simulink model "PID_Simulation_System"  (R2018b)
settings: Solver=VariableStepAuto  StartTime=0.0  StopTime=30  RelTol=1e-3
values from neighbouring files (symbols this model uses):
  h = 5e-3    (= 0.005)    [main.m]
  k_noise = 1    [main.m]
  k_pertub = 1    [main.m]
  kd = 40    [main.m]
  ki = 180    [main.m]
  kp = 497    [main.m]
  p1 = -0.1    [Calc_Aux.m]    (also in main.m = poles(1))
  p2 = poles(2)    [main.m]
  Pertub = 1    [main.m]
  t_pertub = 5    [main.m]
undefined symbols (not defined in the file or in its folder): k
settings Model: Creator=fred  LastModifiedBy=root
settings HardwareCC: ProdBitPerLong=64  ProdHWDeviceType=Intel->x86-64 (Linux 64)

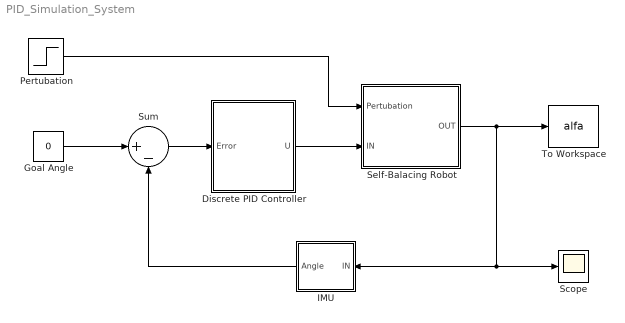
== system PID_Simulation_System ==
  Discrete PID Controller : Subsystem
  Goal Angle : Constant  Value=0
  IMU : Subsystem
  Pertubation : Step  Time=t_pertub  After=Pertub  SampleTime=h
  Scope : Scope
  Self-Balacing Robot : Subsystem
  Sum : Sum  Inputs=|+-
  To Workspace : ToWorkspace  VariableName=alfa  SaveFormat=Timeseries  SampleTime=-1
      settings: Save2DSignal=2-D array (concatenate along first dimension)
  wires:
  Goal Angle/1 -> Sum/1
  IMU/1(Angle) -> Sum/2
  Self-Balacing Robot/1(OUT) -> To Workspace/1, Scope/1, IMU/1(IN)
  Sum/1 -> Discrete PID Controller/1(Error)
  Discrete PID Controller/1(U) -> Self-Balacing Robot/2(IN)
  Pertubation/1 -> Self-Balacing Robot/1(Pertubation)

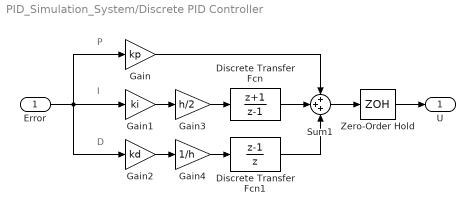
== system PID_Simulation_System/Discrete PID Controller ==
  note: I
  note: D
  note: P
  Error : Inport
  Discrete Transfer Fcn : DiscreteTransferFcn  Numerator=[1 +1]  Denominator=[1 -1]  SampleTime=h
  Discrete Transfer Fcn1 : DiscreteTransferFcn  Numerator=[1 -1]  Denominator=[1 0]  SampleTime=h
  Gain : Gain  Gain=kp
  Gain1 : Gain  Gain=ki
  Gain2 : Gain  Gain=kd
  Gain3 : Gain  Gain=h/2
  Gain4 : Gain  Gain=1/h
  Sum1 : Sum  Inputs=+++
  Zero-Order Hold : ZeroOrderHold  SampleTime=h
  U : Outport
  wires:
  Gain1/1 -> Gain3/1
  Error/1 -> Gain1/1, Gain2/1, Gain/1
  Zero-Order Hold/1 -> U/1
  Sum1/1 -> Zero-Order Hold/1
  Gain2/1 -> Gain4/1
  Gain/1 -> Sum1/1
  Gain3/1 -> Discrete Transfer Fcn/1
  Discrete Transfer Fcn/1 -> Sum1/2
  Gain4/1 -> Discrete Transfer Fcn1/1
  Discrete Transfer Fcn1/1 -> Sum1/3

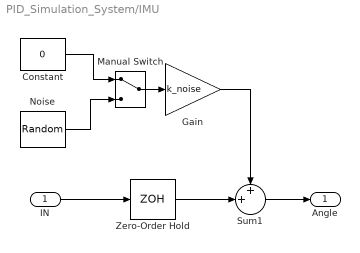
== system PID_Simulation_System/IMU ==
  IN : Inport
  Constant : Constant  Value=0
  Gain : Gain  Gain=k_noise
  Manual Switch : ManualSwitch
  Noise : UniformRandomNumber  Minimum=-0.1  Maximum=0.1  SampleTime=h
  Sum1 : Sum  Inputs=++|
  Zero-Order Hold : ZeroOrderHold  SampleTime=h
  Angle : Outport
  wires:
  IN/1 -> Zero-Order Hold/1
  Constant/1 -> Manual Switch/1
  Noise/1 -> Manual Switch/2
  Manual Switch/1 -> Gain/1
  Gain/1 -> Sum1/1
  Zero-Order Hold/1 -> Sum1/2
  Sum1/1 -> Angle/1

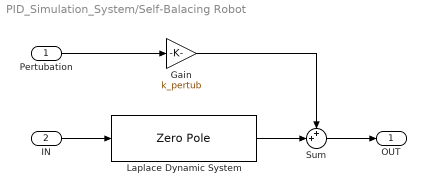
== system PID_Simulation_System/Self-Balacing Robot ==
  Pertubation : Inport
  IN : Inport  Port=2
  Gain : Gain  Gain=k_pertub
  Laplace Dynamic System : ZeroPole  Zeros=[ ]  Poles=[ p1 p2 ]  Gain=k
  Sum : Sum  Inputs=++|
  OUT : Outport
  wires:
  Pertubation/1 -> Gain/1
  Laplace Dynamic System/1 -> Sum/2
  Sum/1 -> OUT/1
  Gain/1 -> Sum/1
  IN/1 -> Laplace Dynamic System/1
